simulink model "Q3b_Simulink"  (R2021a)
settings: Solver=VariableStepAuto  StartTime=0.0  StopTime=2/60  RelTol=1e-3
libraries: fl_lib x19, nesl_utility x10, ee_lib x3, spsFourierLib x2, simulink_extras x1
settings Model: Creator=bemen  LastModifiedBy=bemen

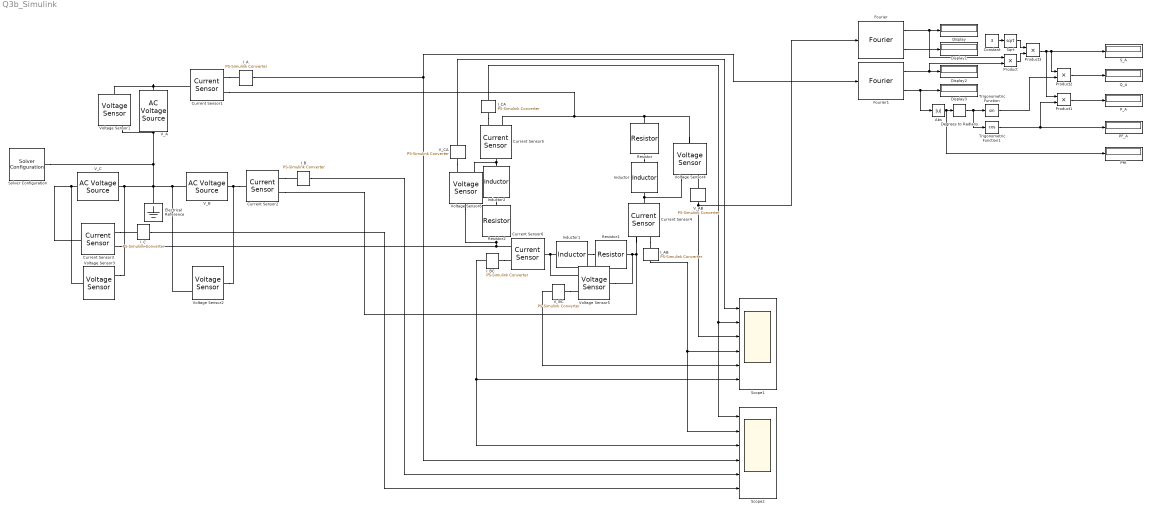
== system Q3b_Simulink ==
  Abs : Abs
  Constant : Constant  Value=3
  Current Sensor{1..6} (6 alike) : fl_lib/Electrical/Electrical Sensors/Current Sensor
  Degrees to Radians : simulink_extras/Transformations/Degrees to Radians
  Display{,1..3} (4 alike) : Display
  Electrical Reference : fl_lib/Electrical/Electrical Elements/Electrical Reference
  Fourier : spsFourierLib/Fourier  Freq=60  n=1  InInit=[0, 0]  Ts=0
      settings: SourceProductBaseCode=PS
  Fourier1 : spsFourierLib/Fourier  Freq=60  n=1  InInit=[0, 0]  Ts=0
      settings: SourceProductBaseCode=PS
  I_A : nesl_utility/PS-Simulink Converter  PhysicalDomain=network_engine_domain  SubClassName=ps_output  LeftPortType=input  RightPortType=output  PseudoPeriodic=off  Frequencies=[]  Unit=inherit  AffineConversion=off
      settings: SourceProductBaseCode=PW,SS
  I_AB : nesl_utility/PS-Simulink Converter  PhysicalDomain=network_engine_domain  SubClassName=ps_output  LeftPortType=input  RightPortType=output  PseudoPeriodic=off  Frequencies=[]  Unit=inherit  AffineConversion=off
      settings: SourceProductBaseCode=PW,SS
  I_B : nesl_utility/PS-Simulink Converter  PhysicalDomain=network_engine_domain  SubClassName=ps_output  LeftPortType=input  RightPortType=output  PseudoPeriodic=off  Frequencies=[]  Unit=inherit  AffineConversion=off
      settings: SourceProductBaseCode=PW,SS
  I_BC : nesl_utility/PS-Simulink Converter  PhysicalDomain=network_engine_domain  SubClassName=ps_output  LeftPortType=input  RightPortType=output  PseudoPeriodic=off  Frequencies=[]  Unit=inherit  AffineConversion=off
      settings: SourceProductBaseCode=PW,SS
  I_C : nesl_utility/PS-Simulink Converter  PhysicalDomain=network_engine_domain  SubClassName=ps_output  LeftPortType=input  RightPortType=output  PseudoPeriodic=off  Frequencies=[]  Unit=inherit  AffineConversion=off
      settings: SourceProductBaseCode=PW,SS
  I_CA : nesl_utility/PS-Simulink Converter  PhysicalDomain=network_engine_domain  SubClassName=ps_output  LeftPortType=input  RightPortType=output  PseudoPeriodic=off  Frequencies=[]  Unit=inherit  AffineConversion=off
      settings: SourceProductBaseCode=PW,SS
  Inductor : fl_lib/Electrical/Electrical Elements/Inductor  l=13.26291192 mH  r=0 Ohm  g=1e-9 1/Ohm  i_specify=off  i_priority=None  i=0 A  i_nominal_specify=off  i_nominal_unit=A  i_nominal_value=1  v_specify=off  v_priority=None  v=0 V  v_nominal_specify=off  v_nominal_unit=V  v_nominal_value=1  i_L_specify=off  i_L_priority=High  i_L=0 A  i_L_nominal_specify=off  i_L_nominal_unit=A  i_L_nominal_value=1
  Inductor1 : fl_lib/Electrical/Electrical Elements/Inductor  l=13.26291192 mH  r=0 Ohm  g=1e-9 1/Ohm  i_specify=off  i_priority=None  i=0 A  i_nominal_specify=off  i_nominal_unit=A  i_nominal_value=1  v_specify=off  v_priority=None  v=0 V  v_nominal_specify=off  v_nominal_unit=V  v_nominal_value=1  i_L_specify=off  i_L_priority=High  i_L=0 A  i_L_nominal_specify=off  i_L_nominal_unit=A  i_L_nominal_value=1
  Inductor2 : fl_lib/Electrical/Electrical Elements/Inductor  l=13.26291192 mH  r=0 Ohm  g=1e-9 1/Ohm  i_specify=off  i_priority=None  i=0 A  i_nominal_specify=off  i_nominal_unit=A  i_nominal_value=1  v_specify=off  v_priority=None  v=0 V  v_nominal_specify=off  v_nominal_unit=V  v_nominal_value=1  i_L_specify=off  i_L_priority=High  i_L=0 A  i_L_nominal_specify=off  i_L_nominal_unit=A  i_L_nominal_value=1
  PF_A : Display
  PHI : Display
  P_A : Display
  Product{,1..3} (4 alike) : Product
  Q_A : Display
  Resistor : ee_lib/Passive/Resistor  R=5 Ohm  R_tol=5  enable_R_tol=0  tol_distribution=1  nSigma=4  enable_operating_limits=0  operating_limit_action=2  max_working_voltage=100 V  power_rating=1 W  enable_faults=0  fault_action=1  R_faulted=inf Ohm  enable_temporal_fault=0  t_fault=1 s  enable_behavioral_fault=0  max_permissible_current=1 A  t_fail_on_current=1 s  noise_mode=0  sample_time=1e-3 s  repeatability=1  auto_seed=272320257  user_seed=0  Tdevice=25 degC  alpha=3.93e-3 1/K  Tmeas=25 degC  thermal_mass=100 J/K  power_derating_T1=70 degC  power_derating_T2=155 degC  operating_temperature_range_vec=[-50, 150] degC  temperature_specify=off  temperature_priority=High  temperature=298.15 K  temperature_nominal_specify=off  temperature_nominal_unit=K  temperature_nominal_value=1
  Resistor1 : ee_lib/Passive/Resistor  R=5 Ohm  R_tol=5  enable_R_tol=0  tol_distribution=1  nSigma=4  enable_operating_limits=0  operating_limit_action=2  max_working_voltage=100 V  power_rating=1 W  enable_faults=0  fault_action=1  R_faulted=inf Ohm  enable_temporal_fault=0  t_fault=1 s  enable_behavioral_fault=0  max_permissible_current=1 A  t_fail_on_current=1 s  noise_mode=0  sample_time=1e-3 s  repeatability=1  auto_seed=2486457467  user_seed=0  Tdevice=25 degC  alpha=3.93e-3 1/K  Tmeas=25 degC  thermal_mass=100 J/K  power_derating_T1=70 degC  power_derating_T2=155 degC  operating_temperature_range_vec=[-50, 150] degC  temperature_specify=off  temperature_priority=High  temperature=298.15 K  temperature_nominal_specify=off  temperature_nominal_unit=K  temperature_nominal_value=1
  Resistor2 : ee_lib/Passive/Resistor  R=5 Ohm  R_tol=5  enable_R_tol=0  tol_distribution=1  nSigma=4  enable_operating_limits=0  operating_limit_action=2  max_working_voltage=100 V  power_rating=1 W  enable_faults=0  fault_action=1  R_faulted=inf Ohm  enable_temporal_fault=0  t_fault=1 s  enable_behavioral_fault=0  max_permissible_current=1 A  t_fail_on_current=1 s  noise_mode=0  sample_time=1e-3 s  repeatability=1  auto_seed=3723251549  user_seed=0  Tdevice=25 degC  alpha=3.93e-3 1/K  Tmeas=25 degC  thermal_mass=100 J/K  power_derating_T1=70 degC  power_derating_T2=155 degC  operating_temperature_range_vec=[-50, 150] degC  temperature_specify=off  temperature_priority=High  temperature=298.15 K  temperature_nominal_specify=off  temperature_nominal_unit=K  temperature_nominal_value=1
  S_A : Display
  Scope1 : Scope  NumInputPorts=6
  Scope2 : Scope  NumInputPorts=6
  Solver Configuration : nesl_utility/Solver Configuration  PhysicalDomain=network_engine_domain  SubClassName=solver  LeftPortType=input  RightPortType=generic  Tones=[]  Harmonics=[]  SimulateNoise=off  Profile=off  UseLocalSampling=off  EnableSwitchedLinearOptims=on  FrequencyDomain=off  UseCCode=off  RelTol=0.001  AbsTol=1e-06  MinStep=1e-09  ToWorkspace=off  RevertToSquareIcSolve=off  NumHomotopyIterations=100  PhasorMode=off  PhasorModeNumHarmonics=1  DoDC=on  ResidualTolerance=1e-09  UseLocalSolver=off  LocalSolverChoice=NE_BACKWARD_EULER_ADVANCER  LocalSolverSampleTime=0.001  DoFixedCost=off  MaxNonlinIter=3  MaxModeIter=2  ComputeImpulses=off  ImpulseIterations=2  LinearAlgebra=auto  EquationFormulation=NE_TIME_EF  DelaysMemoryBudget=1024  AutomaticFiltering=on  FilteringTimeConstant=0.001  PartitionStorageMethod=AS_NEEDED  PartitionMemoryBudget=1024  PartitionMethod=ROBUST
      settings: SourceProductBaseCode=PW,SS
  Sqrt : Sqrt  SaturateOnIntegerOverflow=on
  Trigonometric Function : Trigonometry
  Trigonometric Function1 : Trigonometry  Operator=cos
  V_A : fl_lib/Electrical/Electrical Sources/AC Voltage Source  amp=120 V  shift=0 deg  frequency=60 Hz  omega=0 rad/s
  V_AB : nesl_utility/PS-Simulink Converter  PhysicalDomain=network_engine_domain  SubClassName=ps_output  LeftPortType=input  RightPortType=output  PseudoPeriodic=off  Frequencies=[]  Unit=inherit  AffineConversion=off
      settings: SourceProductBaseCode=PW,SS
  V_B : fl_lib/Electrical/Electrical Sources/AC Voltage Source  amp=120 V  shift=-120 deg  frequency=60 Hz  omega=0 rad/s
  V_BC : nesl_utility/PS-Simulink Converter  PhysicalDomain=network_engine_domain  SubClassName=ps_output  LeftPortType=input  RightPortType=output  PseudoPeriodic=off  Frequencies=[]  Unit=inherit  AffineConversion=off
      settings: SourceProductBaseCode=PW,SS
  V_C : fl_lib/Electrical/Electrical Sources/AC Voltage Source  amp=120 V  shift=120 deg  frequency=60 Hz  omega=0 rad/s
  V_CA : nesl_utility/PS-Simulink Converter  PhysicalDomain=network_engine_domain  SubClassName=ps_output  LeftPortType=input  RightPortType=output  PseudoPeriodic=off  Frequencies=[]  Unit=inherit  AffineConversion=off
      settings: SourceProductBaseCode=PW,SS
  Voltage Sensor{1..6} (6 alike) : fl_lib/Electrical/Electrical Sensors/Voltage Sensor
  wires:
  Fourier/2 -> Display1/1
  Fourier1/1 -> Product/2, Display2/1
  Fourier1/2 -> Abs/1, Display3/1
  Degrees to Radians/1 -> Trigonometric Function1/1, Trigonometric Function/1
  Fourier/1 -> Product/1, Display/1
  Abs/1 -> PHI/1, Degrees to Radians/1
  Constant/1 -> Sqrt/1
  Sqrt/1 -> Product3/1
  Product/1 -> Product3/2
  Product3/1 -> Product1/1, Product2/1, S_A/1
  Trigonometric Function/1 -> Product2/2
  Trigonometric Function1/1 -> Product1/2, PF_A/1
  Product2/1 -> Q_A/1
  Product1/1 -> P_A/1
  V_CA/1 -> Scope1/1
  I_CA/1 -> Scope2/1, Scope1/2
  V_AB/1 -> Fourier/1, Scope1/3
  I_AB/1 -> Scope2/2, Scope1/4
  V_BC/1 -> Scope1/5
  I_BC/1 -> Scope2/3, Scope1/6
  I_A/1 -> Scope2/4, Fourier1/1
  I_B/1 -> Scope2/5
  I_C/1 -> Scope2/6
  connections:
  Resistor/RConn1 -- Inductor/LConn1
  Voltage Sensor3/RConn2 -- V_C/RConn1 -- Electrical Reference/LConn1 -- V_B/RConn1 -- Voltage Sensor2/RConn2 -- Solver Configuration/RConn1 -- Voltage Sensor1/RConn2 -- V_A/RConn1
  V_C/LConn1 -- Voltage Sensor3/LConn1 -- Current Sensor3/LConn1
  V_A/LConn1 -- Current Sensor1/LConn1 -- Voltage Sensor1/LConn1
  Current Sensor2/LConn1 -- V_B/LConn1 -- Voltage Sensor2/LConn1
  Inductor2/LConn1 -- Resistor2/RConn1
  Inductor1/LConn1 -- Resistor1/RConn1
  Resistor1/LConn1 -- Voltage Sensor5/LConn1 -- Current Sensor4/RConn2 -- Current Sensor2/RConn2
  Resistor/LConn1 -- Current Sensor5/RConn2 -- Current Sensor1/RConn2 -- Voltage Sensor4/LConn1
  Current Sensor4/LConn1 -- Voltage Sensor4/RConn2 -- Inductor/RConn1
  Current Sensor3/RConn2 -- Current Sensor6/RConn2 -- Voltage Sensor6/LConn1 -- Resistor2/LConn1
  Current Sensor5/LConn1 -- Voltage Sensor6/RConn2 -- Inductor2/RConn1
  Current Sensor6/LConn1 -- Voltage Sensor5/RConn2 -- Inductor1/RConn1
  I_BC/LConn1 -- Current Sensor6/RConn1
  V_BC/LConn1 -- Voltage Sensor5/RConn1
  V_CA/LConn1 -- Voltage Sensor6/RConn1
  I_CA/LConn1 -- Current Sensor5/RConn1
  V_AB/LConn1 -- Voltage Sensor4/RConn1
  Current Sensor4/RConn1 -- I_AB/LConn1
  Current Sensor3/RConn1 -- I_C/LConn1
  Current Sensor2/RConn1 -- I_B/LConn1
  Current Sensor1/RConn1 -- I_A/LConn1
